simulink model "model_statex_discrete"  (R2016a)
settings: Solver=VariableStepAuto  StartTime=0.0  StopTime=10.0  RelTol=1e-3
values from neighbouring files (symbols this model uses):
  K = place(A, B, Pcom)    [Model_C1.m]
  Nbar = 1    [Model_C1.m]
  Step_final = 4    [Model_C1.m]
  Tech = 0.1    [Model_C1.m]
undefined symbols (not defined in the file or in its folder): Ad, Bd, Cd
settings Model: Creator=massona  LastModifiedBy=massona

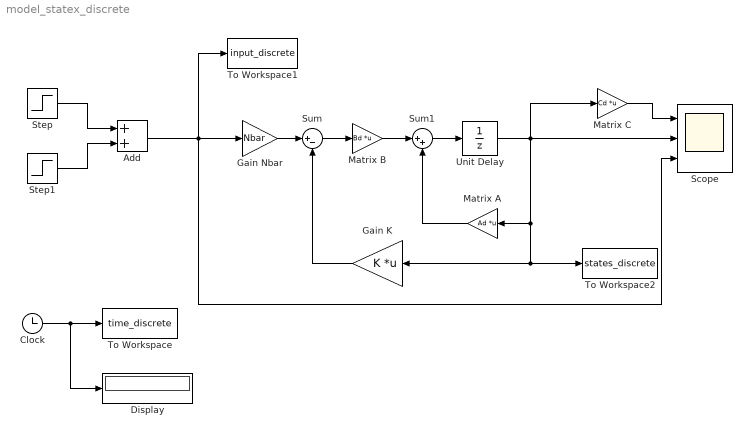
== system model_statex_discrete ==
  Add : Sum
  Clock : Clock
  Display : Display
  Gain K : Gain  Gain=K  Multiplication=Matrix(K*u) (u vector)
  Gain Nbar : Gain  Gain=Nbar
  Matrix A : Gain  Gain=Ad  Multiplication=Matrix(K*u)
  Matrix B : Gain  Gain=Bd  Multiplication=Matrix(K*u)
  Matrix C : Gain  Gain=Cd  Multiplication=Matrix(K*u)
  Scope : Scope  NumInputPorts=3
  Step : Step  After=Step_final  SampleTime=0
  Step1 : Step  Time=6  After=-Step_final  SampleTime=0
  Sum : Sum  Inputs=|+-
  Sum1 : Sum  Inputs=|++
  To Workspace : ToWorkspace  VariableName=time_discrete  SampleTime=Tech
  To Workspace1 : ToWorkspace  VariableName=input_discrete  SampleTime=Tech
  To Workspace2 : ToWorkspace  VariableName=states_discrete  SampleTime=-1
  Unit Delay : UnitDelay  SampleTime=Tech
  wires:
  Step/1 -> Add/1
  Step1/1 -> Add/2
  Clock/1 -> Display/1, To Workspace/1
  Add/1 -> Scope/3, Gain Nbar/1, To Workspace1/1
  Gain Nbar/1 -> Sum/1
  Sum/1 -> Matrix B/1
  Matrix B/1 -> Sum1/1
  Unit Delay/1 -> Matrix C/1, Scope/2, Gain K/1, To Workspace2/1, Matrix A/1
  Matrix A/1 -> Sum1/2
  Gain K/1 -> Sum/2
  Matrix C/1 -> Scope/1
  Sum1/1 -> Unit Delay/1
